simulink model "sm_car"  (R2025b)
settings: Solver=ode23t  StartTime=0.0  StopTime=100  MaxStep=0.4  RelTol=1e-3  AbsTol=1e-3  EnableMultiTasking=on
PreLoadFcn:
  | % Due to usability issue in Repeating Sequence block
  | warning('off','Simulink:Masking:Invalid');
  | 
  | % Eliminate unnecessary warnings in inactive variants
  | % Warnings generated only if you click through inactive variant
  | warning('off','MATLAB:nonExistentField');
  | warning('off','Simulink:Parameters:BlkParamUndefined');
PostLoadFcn:
  | set_param([bdroot '/Vehicle'],'popup_trailer','Off')
  | warning('off','sm:sli:setup:compile:LocalSolverNotSupported')
  | %sm_car_config_maneuver(bdroot,'WOT Braking');
  | sm_car_config_vehicle(bdroot,'false');
  | sm_car_config_logging(bdroot);
InitFcn:
  | sm_car_config_camera;
  | Vehicle = sm_car_vehcfg_checkConfig(Vehicle);
  | sm_car_check_tire_model(bdroot);
StartFcn:
  | tic;
StopFcn:
  | Elapsed_Sim_Time = toc;
  | % disp(['Elapsed Sim Time = ' num2str(Elapsed_Sim_Time)]);
undefined symbols (not defined in the file): Axle1D, AxleIn, Camera, Control, Driver, Init, Maneuver, Pedal, Scene, ShaftL1, ShaftL2, ShaftR1, ShaftR2, Visual, X, xy_data_car_side, Y, Z
libraries: sm_lib x255, fl_lib x191, nesl_utility x149, simulink x23, sdl_lib x14, simulink_extras x8, SimscapeFluids_lib x7, Scene_Utilities x6, Tire_1x2x x4, ee_lib x3, Linkage x2, fuzblock x1
(part 6 of 19)

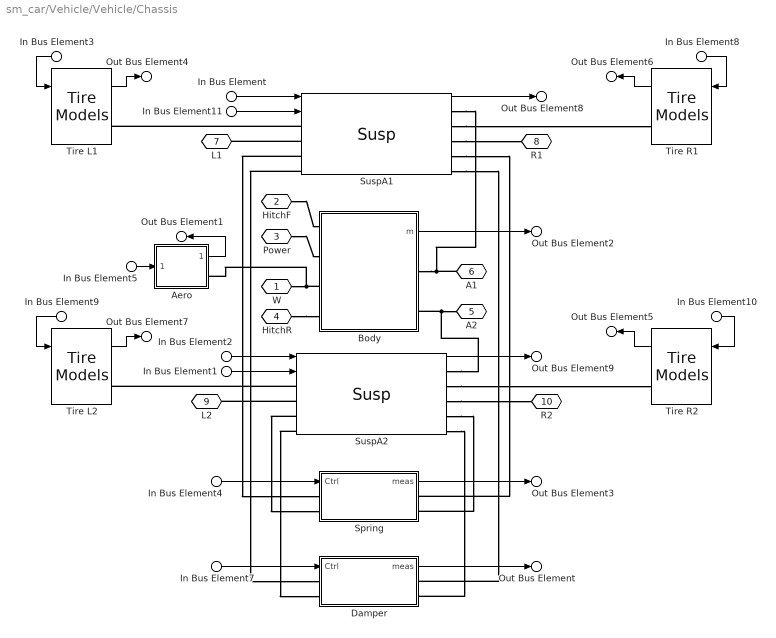
== system sm_car/Vehicle/Vehicle/Chassis ==
  In Bus Element11 : Inport  PortName=DrvBus
  In Bus Element1 : Inport  PortName=DrvBus
  In Bus Element3 : Inport  Port=2  PortName=RdBus  Element=L1
  In Bus Element8 : Inport  Port=2  PortName=RdBus  Element=R1
  In Bus Element10 : Inport  Port=2  PortName=RdBus  Element=R2
  In Bus Element9 : Inport  Port=2  PortName=RdBus  Element=L2
  In Bus Element5 : Inport  Port=2  PortName=RdBus  Element=fWindCar
  In Bus Element7 : Inport  Port=3  PortName=CtrlBus  Element=Damper
  In Bus Element : Inport  Port=3  PortName=CtrlBus  Element=SuspA1
  In Bus Element4 : Inport  Port=3  PortName=CtrlBus  Element=Spring
  In Bus Element2 : Inport  Port=3  PortName=CtrlBus  Element=SuspA2
  Aero : Subsystem  mask(Aerodynamic Load (Drag, Lift)){CL=Chassis.Aero.CL.Value, CD=Chassis.Aero.CD.Value, rho=Chassis.Aero.rho_air.Value, A=Chassis.Aero.ARef.Value, sCentreOfPressure=Chassis.Aero.sPressureCentre.Value, clr_hp=Visual.hp.clr, opc_hp=Visual.hp.opc, rad_hp=Visual.hp.rad}
      mask prompts: CL "Lift Coeff (-)"; CD "Drag Coeff (-)"; rho "Air Density (kg/m^3)"; A "Reference Area (m^2)"; sCentreOfPressure "Centre of Pressure [xyz] (m)"; clr_hp "Color [RGB]"; opc_hp "Opacity (0-1)"; rad_hp "Radius (m)"
      mask help: Models lift and drag on vehicle.
      mask TypeOptions clr_hp:
      | Vis
      | Center of Pressure/GraphicDiffuseColor
      mask TypeOptions opc_hp:
      | Vis
      | Center of Pressure/GraphicOpacity
      mask TypeOptions rad_hp:
      | Vis
      | Center of Pressure/SphereRadius
      mask DialogControl conv_vis Prompt: Visualization
  Body : Subsystem  mask(Body){hp_mount_a1=Chassis.Body.sAxle1.Value, hp_mount_a2=Chassis.Body.sAxle2.Value, hp_mount_power=Chassis.Body.sPower.Value, hp_chassis_cg=Chassis.Body.sCG.Value, hp_mount_hitchf=Chassis.Body.sHitchF.Value, hp_mount_hitchr=Chassis.Body.sHitchR.Value, chassis_mass=Chassis.Body.m.Value, chassis_inertia=Chassis.Body.J.Value, clr_chassis_hp_cg=Visual.hp.clr, opc_chassis_hp_cg=Visual.hp.opc, size_chassis_hp_cg=Visual.hp.rad, BodyGeometry=Chassis.Body.BodyGeometry, BodyLoad=Chassis.Body.BodyLoad}
      mask prompts: hp_mount_power "HP Power [xyz] (m)"; hp_chassis_cg "Chassis CG [xyz] (m)"; hp_mount_hitchf "Hitch Front [xyz] (m)"; hp_mount_hitchr "Hitch Rear [xyz] (m)"; chassis_mass "Mass (kg)"; chassis_inertia "Inertia [Ixx Iyy Izz]"; BodyGeometry "BodyGeometry (structure)"; BodyLoad "BodyLoad (structure)"
      mask help: Vehicle body mass, inertia, and geometry.
      mask TypeOptions hp_mount_a1:
      | Transform
      | Mount A1/TranslationCartesianOffset
      mask TypeOptions hp_mount_a2:
      | Transform
      | Mount A2/TranslationCartesianOffset
      mask TypeOptions hp_mount_power:
      | Transform
      | Power Mount/TranslationCartesianOffset
      mask TypeOptions hp_chassis_cg:
      | Transform
      | Body CG/TranslationCartesianOffset
      mask TypeOptions hp_mount_hitchf:
      | Transform
      | Front Hitch/TranslationCartesianOffset
      mask TypeOptions hp_mount_hitchr:
      | Transform
      | Rear Hitch/TranslationCartesianOffset
      mask TypeOptions chassis_mass:
      | Body Mass
      | and Inertia/Mass
      mask TypeOptions chassis_inertia:
      | Body Mass
      | and Inertia/MomentsOfInertia
      mask TypeOptions clr_chassis_hp_cg:
      | Body Mass
      | and Inertia/GraphicDiffuseColor | Vis HP Mount A1/GraphicDiffuseColor | Vis HP Hitch/GraphicDiffuseColor
      mask TypeOptions opc_chassis_hp_cg:
      | Body Mass
      | and Inertia/GraphicOpacity | Vis HP Mount A1/GraphicOpacity | Vis HP Hitch/GraphicOpacity
      mask TypeOptions size_chassis_hp_cg:
      | Body Mass
      | and Inertia/SphereRadius | Vis HP Mount A1/SphereRadius | Vis HP Hitch/SphereRadius
      mask DialogControl cont_chassis Prompt: Chassis
      mask DialogControl text_chassis_mount_hp_blank Prompt: [xyz] (m)
      mask DialogControl text_chassis_a1 Prompt: Axle 1
      mask DialogControl text_chassis_a2 Prompt: Axle 2
      mask DialogControl text_chassis_hp_mount Prompt: HP Mount
      mask DialogControl cont_chassis_vis Prompt: Visualization
      mask DialogControl text_chassis_vis_clr Prompt: Color [RGB]
      mask DialogControl text_chassis_vis_opc Prompt: Opacity (0-1)
      mask DialogControl text_chassis_vis_size Prompt: Size [xyz] (m)
      mask DialogControl text_chassis_vis_hp Prompt: Hardpoints
      mask DialogControl cont_body_geometry Prompt: Body
      mask Display:
      | % Get image from BodyGeometry.class
      | % (active choice for Body Geometry subsystem)
      | temp_veh_bg_class = lower(get_param([gcb '/Body Geometry'],'LabelModeActiveChoice'));
      | 
      | imagestr = (['sm_car_body_' temp_veh_bg_class '.png']);
      | if(~exist(imagestr))
      |     imagestr = ['sm_car_body_default.png'];
      | end
      | 
      | image(imagestr);
  Damper : Subsystem  Tag=PublishSubsystem  Variant=on  VariantControlMode=label  VariantControl=Variant1  LabelModeActiveChoice=Independent  mask(Variants for Dampers){Damper=Chassis.Damper, VariantLabel=Chassis.Damper.class.Value}
      mask prompts: Damper "Damper Parameters"; VariantLabel "Variant Label"
      mask help: Select option and provide parameters for left and right dampers on two axles. Option is chosen by string provided in Variant Label. The parameters for the selected option is contained in Dampers data structure.
      mask init:
      | curblk = gcb;
      | 
      | % Set variant for this block 
      | set_param(curblk,'LabelModeActiveChoice',VariantLabel);
      settings: AttributesFormatString=%<ActiveVariant>
      mask Display:
      | if(strcmp(get_param(gcb,'LabelModeActiveChoice'),'None'))
      |     disp(' ');
      | else
      |     image('sm_car_vehicle_chassis_damper_IMAGE.png');
      | end
  Spring : Subsystem  Tag=PublishSubsystem  Variant=on  VariantControlMode=label  VariantControl=Variant1  LabelModeActiveChoice=Independent  mask(Variants for Springs){Spring=Chassis.Spring, VariantLabel=Chassis.Spring.class.Value}
      mask prompts: Spring "Spring Parameters"; VariantLabel "Variant Label"
      mask help: Select option and provide parameters for left and right springs on two axles. Option is chosen by string provided in Variant Label. The parameters for the selected option is contained in Springs data structure.
      mask init:
      | curblk = gcb;
      | 
      | % Set variant for this block 
      | set_param(curblk,'LabelModeActiveChoice',VariantLabel);
      settings: AttributesFormatString=%<ActiveVariant>
      mask Display:
      | if(strcmp(get_param(gcb,'LabelModeActiveChoice'),'None'))
      |     disp(' ');
      | else
      |     image('sm_car_vehicle_chassis_spring_IMAGE.png');
      | end
  SuspA1 : Linkage/Susp  VariantControl=Variant1  LabelModeActiveChoice=Linkage  Susp=Chassis.SuspA1  Init=Init.Axle1  VariantLabel=Chassis.SuspA1.class.Value
      settings: AttributesFormatString=%<LabelModeActiveChoice>
  SuspA2 : Linkage/Susp  VariantControl=Variant1  LabelModeActiveChoice=Linkage  Susp=Chassis.SuspA2  Init=Init.Axle2  VariantLabel=Chassis.SuspA2.class.Value
      settings: AttributesFormatString=%<LabelModeActiveChoice>
  Tire L1 : Tire_1x2x/Tire Models  Tag=PublishSubsystem  VariantControl=Variant1  LabelModeActiveChoice=MFEval  popup_leftRight=Left  tir_index=veh_index  Tire=Chassis.Tire  VariantLabel=Chassis.Tire.class.Value
      settings: AttributesFormatString=%<ActiveVariant>
  Tire L2 : Tire_1x2x/Tire Models  Tag=PublishSubsystem  VariantControl=Variant1  LabelModeActiveChoice=MFEval  popup_leftRight=Left  tir_index=veh_index+10  Tire=Chassis.Tire  VariantLabel=Chassis.Tire.class.Value
      settings: AttributesFormatString=%<ActiveVariant>
  Tire R1 : Tire_1x2x/Tire Models  Tag=PublishSubsystem  VariantControl=Variant1  LabelModeActiveChoice=MFEval  popup_leftRight=Right  tir_index=veh_index+4  Tire=Chassis.Tire  VariantLabel=Chassis.Tire.class.Value
      settings: AttributesFormatString=%<ActiveVariant>
  Tire R2 : Tire_1x2x/Tire Models  Tag=PublishSubsystem  VariantControl=Variant1  LabelModeActiveChoice=MFEval  popup_leftRight=Right  tir_index=veh_index+14  Tire=Chassis.Tire  VariantLabel=Chassis.Tire.class.Value
      settings: AttributesFormatString=%<ActiveVariant>
  W : PMIOPort  Side=Right
  HitchF : PMIOPort  Port=2  Side=Right
  Power : PMIOPort  Port=3  Side=Right
  HitchR : PMIOPort  Port=4  Side=Left
  A2 : PMIOPort  Port=5  Side=Right
  A1 : PMIOPort  Port=6  Side=Left
  L1 : PMIOPort  Port=7  Side=Left
  R1 : PMIOPort  Port=8  Side=Right
  L2 : PMIOPort  Port=9  Side=Left
  R2 : PMIOPort  Port=10  Side=Right
  Out Bus Element4 : Outport  VectorParamsAs1DForOutWhenUnconnected=off  PortName=VehBus  Element=WhlL1
  Out Bus Element6 : Outport  VectorParamsAs1DForOutWhenUnconnected=off  PortName=VehBus  Element=WhlR1
  Out Bus Element5 : Outport  VectorParamsAs1DForOutWhenUnconnected=off  PortName=VehBus  Element=WhlR2
  Out Bus Element7 : Outport  VectorParamsAs1DForOutWhenUnconnected=off  PortName=VehBus  Element=WhlL2
  Out Bus Element1 : Outport  VectorParamsAs1DForOutWhenUnconnected=off  PortName=VehBus  Element=Aero
  Out Bus Element : Outport  VectorParamsAs1DForOutWhenUnconnected=off  PortName=VehBus  Element=Damper
  Out Bus Element3 : Outport  VectorParamsAs1DForOutWhenUnconnected=off  PortName=VehBus  Element=Spring
  Out Bus Element8 : Outport  VectorParamsAs1DForOutWhenUnconnected=off  PortName=VehBus  Element=SuspA1
  Out Bus Element9 : Outport  VectorParamsAs1DForOutWhenUnconnected=off  PortName=VehBus  Element=SuspA2
  Out Bus Element2 : Outport  VectorParamsAs1DForOutWhenUnconnected=off  PortName=VehBus  Element=Body
  wires:
  Body/1(m) -> Out Bus Element2/1
  In Bus Element5/1 -> Aero/1(fWind)
  Aero/1(meas) -> Out Bus Element1/1
  In Bus Element4/1 -> Spring/1("Ctrl ")
  In Bus Element7/1 -> Damper/1("Ctrl ")
  In Bus Element2/1 -> SuspA2/1
  SuspA2/1 -> Out Bus Element9/1
  In Bus Element1/1 -> SuspA2/2
  In Bus Element/1 -> SuspA1/1
  SuspA1/1 -> Out Bus Element8/1
  In Bus Element11/1 -> SuspA1/2
  Tire R2/1 -> Out Bus Element5/1
  In Bus Element9/1 -> Tire L2/1
  Tire L1/1 -> Out Bus Element4/1
  In Bus Element8/1 -> Tire R1/1
  Tire L2/1 -> Out Bus Element7/1
  In Bus Element10/1 -> Tire R2/1
  Tire R1/1 -> Out Bus Element6/1
  In Bus Element3/1 -> Tire L1/1
  Damper/1(" meas") -> Out Bus Element/1
  Spring/1(" meas") -> Out Bus Element3/1
  connections:
  HitchR/RConn1 -- Body/LConn4
  Power/RConn1 -- Body/LConn2
  SuspA2/RConn5 -- Damper/RConn2
  SuspA2/LConn4 -- Damper/LConn2
  SuspA2/RConn4 -- Spring/RConn2
  SuspA2/LConn3 -- Spring/LConn2
  SuspA2/RConn3 -- R2/RConn1
  SuspA2/LConn2 -- L2/RConn1
  SuspA2/RConn2 -- Tire R2/RConn1
  SuspA2/LConn1 -- Tire L2/RConn1
  SuspA1/RConn5 -- Damper/RConn1
  SuspA1/LConn4 -- Damper/LConn1
  SuspA1/RConn4 -- Spring/RConn1
  SuspA1/LConn3 -- Spring/LConn1
  Body/RConn1 -- SuspA1/RConn1 -- A1/RConn1
  SuspA1/LConn1 -- Tire L1/RConn1
  SuspA1/RConn2 -- Tire R1/RConn1
  SuspA1/RConn3 -- R1/RConn1
  SuspA1/LConn2 -- L1/RConn1
  A2/RConn1 -- SuspA2/RConn1 -- Body/RConn2
  W/RConn1 -- Aero/RConn1 -- Body/LConn3
  HitchF/RConn1 -- Body/LConn1

== system sm_car/Vehicle/Vehicle/Powertrain ==
  CtrlD : Inport
  CtrlP : Inport  Port=2
  VehB : Inport  Port=3
  Driveline : Subsystem  Tag=PublishSubsystem  Variant=on  VariantControlMode=label  VariantControl=Shaft  LabelModeActiveChoice=L2_R2  mask(Variants for Driveline){Driveline=Powertrain.Driveline, VariantLabel=Powertrain.Driveline.class.Value}
      mask prompts: Driveline "Driveline Parameters"; VariantLabel "Variant Label"
      mask help: Select option and provide parameters for driveline. Option is chosen by string provided in Variant Label. The parameters for the selected option are contained in Driveline data structure.
      mask init:
      | curblk = gcb;
      | 
      | % Set variant for this block 
      | set_param(curblk,'LabelModeActiveChoice',VariantLabel);
      settings: AttributesFormatString=%<ActiveVariant>
      mask Help: web('sm_car_doc_driveline.html');
  Power : Subsystem  Variant=on  VariantControlMode=label  VariantControl=Variant1  LabelModeActiveChoice=Electric_L2_R2  mask(Variants for Power){Power=Powertrain.Power, VariantLabel=Powertrain.Power.class.Value}
      mask prompts: Power "Power Parameters"; VariantLabel "Variant Label"
      mask help: Select option and provide parameters for power system (energy storage and actuator). Option is chosen by string provided in Variant Label. The parameters for the selected option are contained in Power data structure.
      mask init:
      | curblk = gcb;
      | 
      | % Set variant for this block 
      | set_param(curblk,'LabelModeActiveChoice',VariantLabel);
      settings: AttributesFormatString=%<ActiveVariant>
  FA : PMIOPort  Side=Left
  Ref : PMIOPort  Port=2  Side=Right
  RA : PMIOPort  Port=3  Side=Right
  R1 : PMIOPort  Port=4  Side=Right
  L1 : PMIOPort  Port=5  Side=Left
  L2 : PMIOPort  Port=6  Side=Left
  R2 : PMIOPort  Port=7  Side=Right
  OutD : Outport  VectorParamsAs1DForOutWhenUnconnected=off
  OutP : Outport  Port=2  VectorParamsAs1DForOutWhenUnconnected=off
  wires:
  Driveline/1(OutD) -> OutD/1
  CtrlD/1 -> Driveline/1(CtrlBus)
  Power/1(OutP) -> OutP/1
  CtrlP/1 -> Power/1(CtrlBus)
  VehB/1 -> Power/2(VehBus)
  connections:
  Driveline/LConn1 -- FA/RConn1
  Ref/RConn1 -- Power/RConn1
  Driveline/RConn1 -- RA/RConn1
  Driveline/LConn4 -- Power/LConn1
  Driveline/LConn2 -- L1/RConn1
  Driveline/RConn2 -- R1/RConn1
  Driveline/RConn3 -- R2/RConn1
  Driveline/LConn3 -- L2/RConn1

== system sm_car/Vehicle/Vehicle Constraint/No Constraint ==
  F : PMIOPort  Side=Right
  B : PMIOPort  Port=2  Side=Left

== system sm_car/Visualization/Unreal/Animation Off ==
  xyz : Inport
  rpy : Inport  Port=2
  ws : Inport  Port=3
  aCamber : Inport  Port=4
  aSteerWheel : Inport  Port=5
  Terminator{,1..4} (5 alike) : Terminator
  wires:
  rpy/1 -> Terminator1/1
  aSteerWheel/1 -> Terminator4/1
  aCamber/1 -> Terminator3/1
  xyz/1 -> Terminator/1
  ws/1 -> Terminator2/1

== system sm_car/World/Mechanism Configuration/Constant Gravity ==
  MechanismConfiguration : sm_lib/Utilities/Mechanism Configuration  UniformGravity=Constant  GravityVector=GravityVector  GravityVectorUnits=m/s^2  LinearizationDelta=0.001  JointModeTransitionNonlinearIterations=2
  C : PMIOPort  Side=Right
  connections:
  MechanismConfiguration/RConn1 -- C/RConn1

== system sm_car/World/Scene/CRG Hockenheim ==
  Finish Line : Subsystem  mask{post_h=geometry.finish_line.post.height, post_r=geometry.finish_line.post.radius, line_w=geometry.finish_line.post.separation, post_clr=geometry.finish_line.post.clr, post_opc=geometry.finish_line.post.opc, offset_xyz=geometry.finish_line.offset.xyz, offset_yaw=geometry.finish_line.offset.yaw, offset_pitch=geometry.finish_line.offset.pitch, offset_roll=geometry.finish_line.offset.roll}
      mask prompts: post_h "Post Height (m)"; post_r "Post Radius (m)"; line_w "Post Separation (m)"; post_clr "Post Color [R G B] (0-1)"; post_opc "Post Opacity (0-1)"; offset_xyz "Line Offset [x y z] (m)"; offset_yaw "Line Orientation yaw (rad)"; offset_pitch "Line Orientation pitch (rad)"; offset_roll "Line Orientation roll (rad)"
  Ground : Ground
  STL Geometry Centerline : Subsystem  mask{stl_file=geometry.centerline.filename, stl_units=geometry.centerline.fileunits, stl_clr=geometry.centerline.clr, stl_opc=geometry.centerline.opc, stl_x=geometry.centerline.x, stl_y=geometry.centerline.y, stl_z=geometry.centerline.z, stl_yaw=geometry.centerline.yaw, stl_pitch=geometry.centerline.pitch, stl_roll=geometry.centerline.roll}
      mask prompts: stl_file "CAD File"; stl_units "Units"; stl_clr "Color [R G B]"; stl_opc "Opacity (0-1)"; stl_x "Offset x (m)"; stl_y "Offset y (m)"; stl_z "Offset z (m)"; stl_yaw "Offset yaw (rad)"; stl_pitch "Offset pitch (rad)"; stl_roll "Offset roll (rad)"
      mask init:
      | set_param([gcb '/Geometry'],'ExtGeomFileName',stl_file);
      | set_param([gcb '/Geometry'],'ExtGeomFileUnits',stl_units);
  STL Geometry Road : Subsystem  mask{stl_file=geometry.filename, stl_units=geometry.fileunits, stl_clr=geometry.clr, stl_opc=geometry.opc, stl_x=geometry.x, stl_y=geometry.y, stl_z=geometry.z, stl_yaw=geometry.yaw, stl_pitch=geometry.pitch, stl_roll=geometry.roll}
      mask prompts: stl_file "CAD File"; stl_units "Units"; stl_clr "Color [R G B]"; stl_opc "Opacity (0-1)"; stl_x "Offset x (m)"; stl_y "Offset y (m)"; stl_z "Offset z (m)"; stl_yaw "Offset yaw (rad)"; stl_pitch "Offset pitch (rad)"; stl_roll "Offset roll (rad)"
      mask init:
      | set_param([gcb '/Geometry'],'ExtGeomFileName',stl_file);
      | set_param([gcb '/Geometry'],'ExtGeomFileUnits',stl_units);
  W : PMIOPort  Side=Left
  Obs : Outport  VectorParamsAs1DForOutWhenUnconnected=off
  wires:
  Ground/1 -> Obs/1
  connections:
  STL Geometry Centerline/RConn1 -- Finish Line/LConn1 -- W/RConn1 -- STL Geometry Road/RConn1

== system sm_car/World/Scene/CRG Hockenheim F ==
  Finish Line : Subsystem  mask{post_h=geometry.finish_line.post.height, post_r=geometry.finish_line.post.radius, line_w=geometry.finish_line.post.separation, post_clr=geometry.finish_line.post.clr, post_opc=geometry.finish_line.post.opc, offset_xyz=geometry.finish_line.offset.xyz, offset_yaw=geometry.finish_line.offset.yaw, offset_pitch=geometry.finish_line.offset.pitch, offset_roll=geometry.finish_line.offset.roll}
      mask prompts: post_h "Post Height (m)"; post_r "Post Radius (m)"; line_w "Post Separation (m)"; post_clr "Post Color [R G B] (0-1)"; post_opc "Post Opacity (0-1)"; offset_xyz "Line Offset [x y z] (m)"; offset_yaw "Line Orientation yaw (rad)"; offset_pitch "Line Orientation pitch (rad)"; offset_roll "Line Orientation roll (rad)"
  Ground : Ground
  STL Geometry Centerline : Subsystem  mask{stl_file=geometry.centerline.filename, stl_units=geometry.centerline.fileunits, stl_clr=geometry.centerline.clr, stl_opc=geometry.centerline.opc, stl_x=geometry.centerline.x, stl_y=geometry.centerline.y, stl_z=geometry.centerline.z, stl_yaw=geometry.centerline.yaw, stl_pitch=geometry.centerline.pitch, stl_roll=geometry.centerline.roll}
      mask prompts: stl_file "CAD File"; stl_units "Units"; stl_clr "Color [R G B]"; stl_opc "Opacity (0-1)"; stl_x "Offset x (m)"; stl_y "Offset y (m)"; stl_z "Offset z (m)"; stl_yaw "Offset yaw (rad)"; stl_pitch "Offset pitch (rad)"; stl_roll "Offset roll (rad)"
      mask init:
      | set_param([gcb '/Geometry'],'ExtGeomFileName',stl_file);
      | set_param([gcb '/Geometry'],'ExtGeomFileUnits',stl_units);
  STL Geometry Road : Subsystem  mask{stl_file=geometry.filename, stl_units=geometry.fileunits, stl_clr=geometry.clr, stl_opc=geometry.opc, stl_x=geometry.x, stl_y=geometry.y, stl_z=geometry.z, stl_yaw=geometry.yaw, stl_pitch=geometry.pitch, stl_roll=geometry.roll}
      mask prompts: stl_file "CAD File"; stl_units "Units"; stl_clr "Color [R G B]"; stl_opc "Opacity (0-1)"; stl_x "Offset x (m)"; stl_y "Offset y (m)"; stl_z "Offset z (m)"; stl_yaw "Offset yaw (rad)"; stl_pitch "Offset pitch (rad)"; stl_roll "Offset roll (rad)"
      mask init:
      | set_param([gcb '/Geometry'],'ExtGeomFileName',stl_file);
      | set_param([gcb '/Geometry'],'ExtGeomFileUnits',stl_units);
  W : PMIOPort  Side=Left
  Obs : Outport  VectorParamsAs1DForOutWhenUnconnected=off
  wires:
  Ground/1 -> Obs/1
  connections:
  STL Geometry Centerline/RConn1 -- Finish Line/LConn1 -- W/RConn1 -- STL Geometry Road/RConn1

== system sm_car/World/Scene/Double Lane Change ==
  Cones Double Lane Change : Scene_Utilities/Cones Double Lane Change  lane_width=cones.lane_width  lane_separation=cones.lane_lateral_offset  start_lane_a=cones.lane_a_offset  A1_to_A5=cones.lane_a_length  A_to_B_x=cones.gap_a_to_b  B1_to_B5=cones.lane_b_length  B_to_C_x=cones.gap_b_to_c  C1_to_C5=cones.lane_c_length  height=cones.height  baseThickness=cones.base_thickness  baseWidth=cones.base_width  coneBaseDiameter=cones.bottom_diameter  coneTopDiameter=cones.top_diameter  reflectiveStripHeight=cones.strip_height  coneColor=cones.clr  reflectiveStripColor=cones.strip_clr
  Dashes : Scene_Utilities/Dashes  dash_pitch=dashes.pitch  num_dashes=dashes.num  dash_l=dashes.l  dash_h=dashes.h  dash_w=dashes.w  thickness_base=dashes.base_h  dash_clr=dashes.clr  dash_opc=dashes.opc
  Ground : Ground
  Road : Scene_Utilities/Patch Rectangle  gp_l=road.l  gp_w=road.w  gp_h=road.h  gp_clr=road.clr  gp_opc=road.opc
  Transform Cones : sm_lib/Frames and Transforms/Rigid Transform  RotationMethod=None  FollAlignAxisA=+X  BaseAlignAxisA=+Y  FollAlignAxisB=+Y  BaseAlignAxisB=+Z  RotationStandardAxis=+Z  RotationAngle=0.0  RotationAngleUnits=deg  RotationArbitraryAxis=[0 0 1]  RotationSequenceAxes=FollowerAxes  RotationSequence=XYX  RotationSequenceAngles=[0 0 0]  RotationSequenceAnglesUnits=deg  RotationMatrix=[1 0 0; 0 1 0; 0 0 1]  Quaternion=[1 0 0 0]  TranslationMethod=StandardAxis  TranslationCartesianOffset=[0 0 0]  TranslationCartesianOffsetUnits=m  TranslationStandardAxis=-X  TranslationStandardOffset=road.l/2  TranslationStandardOffsetUnits=m  TranslationROffset=0  TranslationROffsetUnits=m  TranslationThetaOffset=0  TranslationThetaOffsetUnits=deg  TranslationZOffset=0  TranslationZOffsetUnits=m
  Transform Road : sm_lib/Frames and Transforms/Rigid Transform  RotationMethod=RotationSequence  FollAlignAxisA=+X  BaseAlignAxisA=+Y  FollAlignAxisB=+Y  BaseAlignAxisB=+Z  RotationStandardAxis=+Z  RotationAngle=0.0  RotationAngleUnits=deg  RotationArbitraryAxis=[0 0 1]  RotationSequenceAxes=BaseAxes  RotationSequence=ZYX  RotationSequenceAngles=[road.yaw road.pitch road.roll]  RotationSequenceAnglesUnits=rad  RotationMatrix=[1 0 0; 0 1 0; 0 0 1]  Quaternion=[1 0 0 0]  TranslationMethod=Cartesian  TranslationCartesianOffset=[road.x road.y road.z]  TranslationCartesianOffsetUnits=m  TranslationStandardAxis=+Z  TranslationStandardOffset=0  TranslationStandardOffsetUnits=m  TranslationROffset=0  TranslationROffsetUnits=m  TranslationThetaOffset=0  TranslationThetaOffsetUnits=deg  TranslationZOffset=0  TranslationZOffsetUnits=m
  W : PMIOPort  Side=Left
  Obs : Outport  VectorParamsAs1DForOutWhenUnconnected=off
  wires:
  Ground/1 -> Obs/1
  connections:
  W/RConn1 -- Transform Road/LConn1
  Dashes/LConn1 -- Road/RConn1 -- Transform Cones/LConn1 -- Transform Road/RConn1
  Cones Double Lane Change/LConn1 -- Transform Cones/RConn1

== system sm_car/World/Scene/Double Lane Change ISO3888 ==
  Cones Double Lane Change : Scene_Utilities/Cones Double Lane Change  lane_width=cones.lane_width  lane_separation=cones.lane_lateral_offset  start_lane_a=cones.lane_a_offset  A1_to_A5=cones.lane_a_length  A_to_B_x=cones.gap_a_to_b  B1_to_B5=cones.lane_b_length  B_to_C_x=cones.gap_b_to_c  C1_to_C5=cones.lane_c_length  height=cones.height  baseThickness=cones.base_thickness  baseWidth=cones.base_width  coneBaseDiameter=cones.bottom_diameter  coneTopDiameter=cones.top_diameter  reflectiveStripHeight=cones.strip_height  coneColor=cones.clr  reflectiveStripColor=cones.strip_clr
  Dashes : Scene_Utilities/Dashes  dash_pitch=dashes.pitch  num_dashes=dashes.num  dash_l=dashes.l  dash_h=dashes.h  dash_w=dashes.w  thickness_base=dashes.base_h  dash_clr=dashes.clr  dash_opc=dashes.opc
  Ground : Ground
  Road : Scene_Utilities/Patch Rectangle  gp_l=road.l  gp_w=road.w  gp_h=road.h  gp_clr=road.clr  gp_opc=road.opc
  Transform Cones : sm_lib/Frames and Transforms/Rigid Transform  RotationMethod=None  FollAlignAxisA=+X  BaseAlignAxisA=+Y  FollAlignAxisB=+Y  BaseAlignAxisB=+Z  RotationStandardAxis=+Z  RotationAngle=0.0  RotationAngleUnits=deg  RotationArbitraryAxis=[0 0 1]  RotationSequenceAxes=FollowerAxes  RotationSequence=XYX  RotationSequenceAngles=[0 0 0]  RotationSequenceAnglesUnits=deg  RotationMatrix=[1 0 0; 0 1 0; 0 0 1]  Quaternion=[1 0 0 0]  TranslationMethod=StandardAxis  TranslationCartesianOffset=[0 0 0]  TranslationCartesianOffsetUnits=m  TranslationStandardAxis=-X  TranslationStandardOffset=road.l/2  TranslationStandardOffsetUnits=m  TranslationROffset=0  TranslationROffsetUnits=m  TranslationThetaOffset=0  TranslationThetaOffsetUnits=deg  TranslationZOffset=0  TranslationZOffsetUnits=m
  Transform Road : sm_lib/Frames and Transforms/Rigid Transform  RotationMethod=RotationSequence  FollAlignAxisA=+X  BaseAlignAxisA=+Y  FollAlignAxisB=+Y  BaseAlignAxisB=+Z  RotationStandardAxis=+Z  RotationAngle=0.0  RotationAngleUnits=deg  RotationArbitraryAxis=[0 0 1]  RotationSequenceAxes=BaseAxes  RotationSequence=ZYX  RotationSequenceAngles=[road.yaw road.pitch road.roll]  RotationSequenceAnglesUnits=rad  RotationMatrix=[1 0 0; 0 1 0; 0 0 1]  Quaternion=[1 0 0 0]  TranslationMethod=Cartesian  TranslationCartesianOffset=[road.x road.y road.z]  TranslationCartesianOffsetUnits=m  TranslationStandardAxis=+Z  TranslationStandardOffset=0  TranslationStandardOffsetUnits=m  TranslationROffset=0  TranslationROffsetUnits=m  TranslationThetaOffset=0  TranslationThetaOffsetUnits=deg  TranslationZOffset=0  TranslationZOffsetUnits=m
  W : PMIOPort  Side=Left
  Obs : Outport  VectorParamsAs1DForOutWhenUnconnected=off
  wires:
  Ground/1 -> Obs/1
  connections:
  W/RConn1 -- Transform Road/LConn1
  Dashes/LConn1 -- Road/RConn1 -- Transform Cones/LConn1 -- Transform Road/RConn1
  Cones Double Lane Change/LConn1 -- Transform Cones/RConn1

== system sm_car/World/Scene/Plane Grid ==
  Grid : Subsystem  mask{grid_x=plane.l, grid_y=plane.w, grid_z=plane.h, grid_line_width=grid.line_width, grid_num_sq_x=grid.num_sqrs_x, grid_num_sq_y=grid.num_sqrs_y, grid_clr=grid.clr, grid_opc=grid.opc}
      mask prompts: grid_x "Length (m) (Global x)"; grid_y "Width (m) (Global y)"; grid_z "Depth (m) (Global z)"; grid_line_width "Line width (m)"; grid_num_sq_x "Number of squares in x"; grid_num_sq_y "Number of squares in y"; grid_clr "Color [RGB]"; grid_opc "Opacity (0-1)"
      mask init:
      | % Derived parameters - for two perpendicular grids with num_sq-by-1 holes
      | % **Note, not num_sq_x by num_sq_y holes - better render speed with
      | % separate meshes for x and y.
      | 
      | hole_lx = (grid_x-(grid_line_width*(grid_num_sq_x+1)))/grid_num_sq_x;
      | hole_wx = (grid_y-(grid_line_width*(1+1)))/1;
      | 
      | hole_ly = (grid_y-(grid_line_width*(grid_num_sq_y+1)))/grid_num_sq_y;
      | hole_wy = (grid_x-(grid_line_width*(1+1)))/1;
  Ground : Ground
  Ground Plane : Subsystem  mask{gp_l=plane.l, gp_w=plane.w, gp_h=plane.h, gp_clr=plane.clr, gp_opc=plane.opc}
      mask prompts: gp_l "Length (m) (Global  x)"; gp_w "Width (m) (Global  y)"; gp_h "Depth (m) (Global z)"; gp_clr "Color [R G B]"; gp_opc "Opacity (0-1)"
  Transform Plane : sm_lib/Frames and Transforms/Rigid Transform  RotationMethod=None  FollAlignAxisA=+X  BaseAlignAxisA=+Y  FollAlignAxisB=+Y  BaseAlignAxisB=+Z  RotationStandardAxis=+Z  RotationAngle=0.0  RotationAngleUnits=deg  RotationArbitraryAxis=[0 0 1]  RotationSequenceAxes=FollowerAxes  RotationSequence=XYX  RotationSequenceAngles=[0 0 0]  RotationSequenceAnglesUnits=deg  RotationMatrix=[1 0 0; 0 1 0; 0 0 1]  Quaternion=[1 0 0 0]  TranslationMethod=Cartesian  TranslationCartesianOffset=[plane.x plane.y plane.z]  TranslationCartesianOffsetUnits=m  TranslationStandardAxis=+Z  TranslationStandardOffset=0  TranslationStandardOffsetUnits=m  TranslationROffset=0  TranslationROffsetUnits=m  TranslationThetaOffset=0  TranslationThetaOffsetUnits=deg  TranslationZOffset=0  TranslationZOffsetUnits=m
  W : PMIOPort  Side=Left
  Obs : Outport  VectorParamsAs1DForOutWhenUnconnected=off
  wires:
  Ground/1 -> Obs/1
  connections:
  Ground Plane/RConn1 -- Transform Plane/RConn1 -- Grid/LConn1
  Transform Plane/LConn1 -- W/RConn1

== system sm_car/World/Scene/Skidpad ==
  Circle Inner L : Subsystem  mask{circ_d=circ_in.d, circ_a1=-180, circ_a2=180, circ_w=circ_in.w, circ_h=circ_in.h, circ_clr=circ_in.clr, circ_opc=circ_in.opc}
      mask prompts: circ_d "Circle Diameter (m)"; circ_a1 "Start Angle (deg)"; circ_a2 "Finish Angle (deg)"; circ_w "Stripe Width (m)"; circ_h "Stripe Height (m)"; circ_clr "Color [RGB]"; circ_opc "Opacity (0-1)"
      mask init:
      | xy_data_circ = Extr_Data_Ring(...
      |     circ_d/2+circ_w/2,circ_d/2-circ_w/2,circ_a1, circ_a2);
  Circle Inner R : Subsystem  mask{circ_d=circ_in.d, circ_a1=-180, circ_a2=180, circ_w=circ_in.w, circ_h=circ_in.h, circ_clr=circ_in.clr, circ_opc=circ_in.opc}
      mask prompts: circ_d "Circle Diameter (m)"; circ_a1 "Start Angle (deg)"; circ_a2 "Finish Angle (deg)"; circ_w "Stripe Width (m)"; circ_h "Stripe Height (m)"; circ_clr "Color [RGB]"; circ_opc "Opacity (0-1)"
      mask init:
      | xy_data_circ = Extr_Data_Ring(...
      |     circ_d/2+circ_w/2,circ_d/2-circ_w/2,circ_a1, circ_a2);
  Circle Outer L : Subsystem  mask{circ_d=circ_out.d, circ_a1=circ_out.ang1, circ_a2=circ_out.ang2, circ_w=circ_out.w, circ_h=circ_out.h, circ_clr=circ_out.clr, circ_opc=circ_out.opc}
      mask prompts: circ_d "Circle Diameter (m)"; circ_a1 "Start Angle (deg)"; circ_a2 "Finish Angle (deg)"; circ_w "Stripe Width (m)"; circ_h "Stripe Height (m)"; circ_clr "Color [RGB]"; circ_opc "Opacity (0-1)"
      mask init:
      | xy_data_circ = Extr_Data_Ring(...
      |     circ_d/2+circ_w/2,circ_d/2-circ_w/2,circ_a1, circ_a2);
  Circle Outer R : Subsystem  mask{circ_d=circ_out.d, circ_a1=circ_out.ang1, circ_a2=circ_out.ang2, circ_w=circ_out.w, circ_h=circ_out.h, circ_clr=circ_out.clr, circ_opc=circ_out.opc}
      mask prompts: circ_d "Circle Diameter (m)"; circ_a1 "Start Angle (deg)"; circ_a2 "Finish Angle (deg)"; circ_w "Stripe Width (m)"; circ_h "Stripe Height (m)"; circ_clr "Color [RGB]"; circ_opc "Opacity (0-1)"
      mask init:
      | xy_data_circ = Extr_Data_Ring(...
      |     circ_d/2+circ_w/2,circ_d/2-circ_w/2,circ_a1, circ_a2);
  Ground : Ground
  Ground Plane : Subsystem  mask{gp_l=plane.l, gp_w=plane.w, gp_h=plane.h, gp_clr=plane.clr, gp_opc=plane.opc}
      mask prompts: gp_l "Length (m) (Global  x)"; gp_w "Width (m) (Global  y)"; gp_h "Depth (m) (Global z)"; gp_clr "Color [R G B]"; gp_opc "Opacity (0-1)"
  Transform Circle L : sm_lib/Frames and Transforms/Rigid Transform  RotationMethod=None  FollAlignAxisA=+X  BaseAlignAxisA=+Y  FollAlignAxisB=+Y  BaseAlignAxisB=+Z  RotationStandardAxis=+Z  RotationAngle=0.0  RotationAngleUnits=deg  RotationArbitraryAxis=[0 0 1]  RotationSequenceAxes=FollowerAxes  RotationSequence=XYX  RotationSequenceAngles=[0 0 0]  RotationSequenceAnglesUnits=deg  RotationMatrix=[1 0 0; 0 1 0; 0 0 1]  Quaternion=[1 0 0 0]  TranslationMethod=Cartesian  TranslationCartesianOffset=[0 circ_in.sep/2 0]  TranslationCartesianOffsetUnits=m  TranslationStandardAxis=+Z  TranslationStandardOffset=0  TranslationStandardOffsetUnits=m  TranslationROffset=0  TranslationROffsetUnits=m  TranslationThetaOffset=0  TranslationThetaOffsetUnits=deg  TranslationZOffset=0  TranslationZOffsetUnits=m
  Transform Circle R : sm_lib/Frames and Transforms/Rigid Transform  RotationMethod=None  FollAlignAxisA=+X  BaseAlignAxisA=+Y  FollAlignAxisB=+Y  BaseAlignAxisB=+Z  RotationStandardAxis=+Z  RotationAngle=0.0  RotationAngleUnits=deg  RotationArbitraryAxis=[0 0 1]  RotationSequenceAxes=FollowerAxes  RotationSequence=XYX  RotationSequenceAngles=[0 0 0]  RotationSequenceAnglesUnits=deg  RotationMatrix=[1 0 0; 0 1 0; 0 0 1]  Quaternion=[1 0 0 0]  TranslationMethod=Cartesian  TranslationCartesianOffset=[0 -circ_in.sep/2 0]  TranslationCartesianOffsetUnits=m  TranslationStandardAxis=+Z  TranslationStandardOffset=0  TranslationStandardOffsetUnits=m  TranslationROffset=0  TranslationROffsetUnits=m  TranslationThetaOffset=0  TranslationThetaOffsetUnits=deg  TranslationZOffset=0  TranslationZOffsetUnits=m
  Transform Orient OuterL : sm_lib/Frames and Transforms/Rigid Transform  RotationMethod=StandardAxis  FollAlignAxisA=+X  BaseAlignAxisA=+Y  FollAlignAxisB=+Y  BaseAlignAxisB=+Z  RotationStandardAxis=+Z  RotationAngle=90  RotationAngleUnits=deg  RotationArbitraryAxis=[0 0 1]  RotationSequenceAxes=FollowerAxes  RotationSequence=XYX  RotationSequenceAngles=[0 0 0]  RotationSequenceAnglesUnits=deg  RotationMatrix=[1 0 0; 0 1 0; 0 0 1]  Quaternion=[1 0 0 0]  TranslationMethod=None  TranslationCartesianOffset=[0 0 0]  TranslationCartesianOffsetUnits=m  TranslationStandardAxis=+Z  TranslationStandardOffset=0  TranslationStandardOffsetUnits=m  TranslationROffset=0  TranslationROffsetUnits=m  TranslationThetaOffset=0  TranslationThetaOffsetUnits=deg  TranslationZOffset=0  TranslationZOffsetUnits=m
  Transform Orient OuterR : sm_lib/Frames and Transforms/Rigid Transform  RotationMethod=StandardAxis  FollAlignAxisA=+X  BaseAlignAxisA=+Y  FollAlignAxisB=+Y  BaseAlignAxisB=+Z  RotationStandardAxis=+Z  RotationAngle=-90  RotationAngleUnits=deg  RotationArbitraryAxis=[0 0 1]  RotationSequenceAxes=FollowerAxes  RotationSequence=XYX  RotationSequenceAngles=[0 0 0]  RotationSequenceAnglesUnits=deg  RotationMatrix=[1 0 0; 0 1 0; 0 0 1]  Quaternion=[1 0 0 0]  TranslationMethod=None  TranslationCartesianOffset=[0 0 0]  TranslationCartesianOffsetUnits=m  TranslationStandardAxis=+Z  TranslationStandardOffset=0  TranslationStandardOffsetUnits=m  TranslationROffset=0  TranslationROffsetUnits=m  TranslationThetaOffset=0  TranslationThetaOffsetUnits=deg  TranslationZOffset=0  TranslationZOffsetUnits=m
  Transform Plane : sm_lib/Frames and Transforms/Rigid Transform  RotationMethod=None  FollAlignAxisA=+X  BaseAlignAxisA=+Y  FollAlignAxisB=+Y  BaseAlignAxisB=+Z  RotationStandardAxis=+Z  RotationAngle=0.0  RotationAngleUnits=deg  RotationArbitraryAxis=[0 0 1]  RotationSequenceAxes=FollowerAxes  RotationSequence=XYX  RotationSequenceAngles=[0 0 0]  RotationSequenceAnglesUnits=deg  RotationMatrix=[1 0 0; 0 1 0; 0 0 1]  Quaternion=[1 0 0 0]  TranslationMethod=Cartesian  TranslationCartesianOffset=[plane.x plane.y plane.z]  TranslationCartesianOffsetUnits=m  TranslationStandardAxis=+Z  TranslationStandardOffset=0  TranslationStandardOffsetUnits=m  TranslationROffset=0  TranslationROffsetUnits=m  TranslationThetaOffset=0  TranslationThetaOffsetUnits=deg  TranslationZOffset=0  TranslationZOffsetUnits=m
  W : PMIOPort  Side=Left
  Obs : Outport  VectorParamsAs1DForOutWhenUnconnected=off
  wires:
  Ground/1 -> Obs/1
  connections:
  Circle Outer L/RConn1 -- Transform Orient OuterL/RConn1
  Circle Outer R/RConn1 -- Transform Orient OuterR/RConn1
  Circle Inner R/RConn1 -- Transform Circle R/RConn1 -- Transform Orient OuterR/LConn1
  Transform Plane/RConn1 -- Ground Plane/RConn1
  Transform Circle L/LConn1 -- W/RConn1 -- Transform Plane/LConn1 -- Transform Circle R/LConn1
  Circle Inner L/RConn1 -- Transform Circle L/RConn1 -- Transform Orient OuterL/LConn1

== system sm_car/Controller/Default/Brake Control/Pedal ==
  rBrakePedal : Inport
  VehBus : Inport  Port=2
  Apply{,1..3} (4 alike) : Constant  Value=[0 1]
  Bus Creator : BusCreator  Inputs=1
  Bus Creator1 : BusCreator  Inputs=4
  Terminator : Terminator
  Terminator1 : Terminator
  Brakes : Outport  VectorParamsAs1DForOutWhenUnconnected=off
  wires:
  rBrakePedal/1 -> Terminator1/1
  Apply3/1 -> Bus Creator1/4  "R2"
  Apply2/1 -> Bus Creator1/3  "L2"
  Apply1/1 -> Bus Creator1/2  "R1"
  Apply/1 -> Bus Creator1/1  "L1"
  Bus Creator1/1 -> Bus Creator/1  "Valves"
  VehBus/1 -> Terminator/1
  Bus Creator/1 -> Brakes/1  "Brakes"

== system sm_car/Controller/FeedF_Ctrl/Brake Control/Pedal ==
  rBrakePedal : Inport
  VehBus : Inport  Port=2
  Apply{,1..3} (4 alike) : Constant  Value=[0 1]
  Bus Creator : BusCreator  Inputs=1
  Bus Creator1 : BusCreator  Inputs=4
  Terminator : Terminator
  Terminator1 : Terminator
  Brakes : Outport  VectorParamsAs1DForOutWhenUnconnected=off
  wires:
  Bus Creator/1 -> Brakes/1  "Brakes"
  VehBus/1 -> Terminator/1
  Bus Creator1/1 -> Bus Creator/1  "Valves"
  Apply/1 -> Bus Creator1/1  "L1"
  Apply1/1 -> Bus Creator1/2  "R1"
  Apply2/1 -> Bus Creator1/3  "L2"
  Apply3/1 -> Bus Creator1/4  "R2"
  rBrakePedal/1 -> Terminator1/1

== system sm_car/Controller/NoIMU/Brake Control/Pedal ==
  rBrakePedal : Inport
  VehBus : Inport  Port=2
  Apply{,1..3} (4 alike) : Constant  Value=[0 1]
  Bus Creator : BusCreator  Inputs=1
  Bus Creator1 : BusCreator  Inputs=4
  Terminator : Terminator
  Terminator1 : Terminator
  Brakes : Outport  VectorParamsAs1DForOutWhenUnconnected=off
  wires:
  Bus Creator/1 -> Brakes/1  "Brakes"
  VehBus/1 -> Terminator/1
  Bus Creator1/1 -> Bus Creator/1  "Valves"
  Apply/1 -> Bus Creator1/1  "L1"
  Apply1/1 -> Bus Creator1/2  "R1"
  Apply2/1 -> Bus Creator1/3  "L2"
  Apply3/1 -> Bus Creator1/4  "R2"
  rBrakePedal/1 -> Terminator1/1

== system sm_car/Controller/NoIMU/Power Control/Current-Torque ==
  note: modify to accomade all voltage ranges
      | only 220V now
  note: current - torque
  V : Inport
  Il : Inport  Port=2
  Ir : Inport  Port=3
  Add : Sum
  Km : Gain  Gain=Km
  Km1 : Gain  Gain=Km
  Terminator : Terminator
  Out1 : Outport
  wires:
  Il/1 -> Km1/1
  Km1/1 -> Add/1
  V/1 -> Terminator/1
  Ir/1 -> Km/1
  Add/1 -> Out1/1
  Km/1 -> Add/2

== system sm_car/Controller/NoIMU/Power Control/Slip Control ==
  VehBus : Inport
  Bus Selector : BusSelector  OutputSignals=Power.MotorL2.w,Power.MotorL2.i,Power.MotorR2.w,Power.MotorR2.i
  Constant : Constant
  Constant1 : Constant  Value=0
  I no load : Constant  Value=I0
  Product : Product
  Product1 : Product
  Relational Operator : RelationalOperator  OutDataTypeStr=boolean  RndMeth=Simplest  InputSameDT=off
  Relational Operator1 : RelationalOperator  Operator=<=  OutDataTypeStr=boolean  RndMeth=Simplest  InputSameDT=off
  Relational Operator2 : RelationalOperator  OutDataTypeStr=boolean  RndMeth=Simplest  InputSameDT=off
  Relational Operator3 : RelationalOperator  Operator=<=  OutDataTypeStr=boolean  RndMeth=Simplest  InputSameDT=off
  Switch : Switch  Criteria=u2 > Threshold  SaturateOnIntegerOverflow=off  InputSameDT=off
  Switch1 : Switch  Criteria=u2 > Threshold  SaturateOnIntegerOverflow=off  InputSameDT=off
  w no load : Constant  Value=w0
  Out1 : Outport
  Out2 : Outport  Port=2
  wires:
  VehBus/1 -> Bus Selector/1
  Bus Selector/1 -> Relational Operator/1  "<w>"
  Product/1 -> Switch/2
  Relational Operator/1 -> Product/1
  Relational Operator1/1 -> Product/2
  Relational Operator2/1 -> Product1/1
  Relational Operator3/1 -> Product1/2
  Product1/1 -> Switch1/2
  Constant1/1 -> Switch/3, Switch1/3
  Constant/1 -> Switch1/1, Switch/1
  Bus Selector/2 -> Relational Operator1/1  "<i>"
  Bus Selector/3 -> Relational Operator2/1  "<w>"
  Bus Selector/4 -> Relational Operator3/1  "<i>"
  I no load/1 -> Relational Operator1/2, Relational Operator3/2
  w no load/1 -> Relational Operator/2, Relational Operator2/2
  Switch/1 -> Out1/1
  Switch1/1 -> Out2/1

== system sm_car/Controller/Slip_Ctrl/Brake Control/Pedal ==
  rBrakePedal : Inport
  VehBus : Inport  Port=2
  Apply{,1..3} (4 alike) : Constant  Value=[0 1]
  Bus Creator : BusCreator  Inputs=1
  Bus Creator1 : BusCreator  Inputs=4
  Terminator : Terminator
  Terminator1 : Terminator
  Brakes : Outport  VectorParamsAs1DForOutWhenUnconnected=off
  wires:
  Bus Creator/1 -> Brakes/1  "Brakes"
  VehBus/1 -> Terminator/1
  Bus Creator1/1 -> Bus Creator/1  "Valves"
  Apply/1 -> Bus Creator1/1  "L1"
  Apply1/1 -> Bus Creator1/2  "R1"
  Apply2/1 -> Bus Creator1/3  "L2"
  Apply3/1 -> Bus Creator1/4  "R2"
  rBrakePedal/1 -> Terminator1/1

== system sm_car/Controller/TrqVec 4Motor/Brake Control/ABS ==
  rBrakePedal : Inport
  In Bus Element1 : Inport  Port=2  PortName=VehBus  Element=Chassis
  In Bus Element2 : Inport  Port=2  PortName=VehBus  Element=Chassis.Body.CG
  Bus Creator1 : BusCreator  Inputs=4
  Bus Creator2 : BusCreator  Inputs=1
  Bus Selector : BusSelector  OutputSignals=L1
  Bus Selector1 : BusSelector  OutputSignals=R1
  Bus Selector2 : BusSelector  OutputSignals=L2
  Bus Selector3 : BusSelector  OutputSignals=R2
  Calculate Slip : Subsystem
  Sensor : Subsystem
  Terminator : Terminator
  Valve Control L1 : Subsystem
  Valve Control L2 : Subsystem
  Valve Control R1 : Subsystem
  Valve Control R2 : Subsystem
  Vehicle Speed : Subsystem
  Brakes : Outport  VectorParamsAs1DForOutWhenUnconnected=off
  wires:
  rBrakePedal/1 -> Terminator/1
  Vehicle Speed/1(vSpdEst) -> Valve Control R2/2(vSpdEst), Valve Control L2/2(vSpdEst), Valve Control R1/2(vSpdEst), Valve Control L1/2(vSpdEst), Calculate Slip/2(VehSpdEst)
  Sensor/1(GroundSpd) -> Vehicle Speed/1(Sensors), Calculate Slip/1(WhlSpd)
  Bus Creator1/1 -> Bus Creator2/1  "Valves"
  Bus Selector2/1 -> Valve Control L2/1(Slip)  "<L2>"
  Valve Control R1/1(Valve) -> Bus Creator1/2  "R1"
  Valve Control R2/1(Valve) -> Bus Creator1/4  "R2"
  Valve Control L2/1(Valve) -> Bus Creator1/3  "L2"
  Bus Selector3/1 -> Valve Control R2/1(Slip)  "<R2>"
  Bus Selector/1 -> Valve Control L1/1(Slip)  "<L1>"
  Calculate Slip/1(Slip) -> Bus Selector3/1, Bus Selector2/1, Bus Selector1/1, Bus Selector/1
  Valve Control L1/1(Valve) -> Bus Creator1/1  "L1"
  Bus Selector1/1 -> Valve Control R1/1(Slip)  "<R1>"
  Bus Creator2/1 -> Brakes/1  "Brakes"
  In Bus Element1/1 -> Sensor/2(WhlSpd)
  In Bus Element2/1 -> Sensor/1(Body)

== system sm_car/Controller/TrqVec 4Motor/Brake Control/Pedal ==
  rBrakePedal : Inport
  VehBus : Inport  Port=2
  Apply{,1..3} (4 alike) : Constant  Value=[0 1]
  Bus Creator : BusCreator  Inputs=1
  Bus Creator1 : BusCreator  Inputs=4
  Terminator : Terminator
  Terminator1 : Terminator
  Brakes : Outport  VectorParamsAs1DForOutWhenUnconnected=off
  wires:
  rBrakePedal/1 -> Terminator1/1
  Apply3/1 -> Bus Creator1/4  "R2"
  Apply2/1 -> Bus Creator1/3  "L2"
  Apply1/1 -> Bus Creator1/2  "R1"
  Apply/1 -> Bus Creator1/1  "L1"
  Bus Creator1/1 -> Bus Creator/1  "Valves"
  VehBus/1 -> Terminator/1
  Bus Creator/1 -> Brakes/1  "Brakes"

== system sm_car/Controller/TrqVec 4Motor/Brake Control/Pressure ==
  rBrakePedal : Inport
  VehBus : Inport  Port=2
  Bus Creator : BusCreator  Inputs=4
  Gain : Gain  Gain=Vehicle.Brakes.Front.Caliper.pMax.Value
  Gain1 : Gain  Gain=Vehicle.Brakes.Front.Caliper.pMax.Value
  Gain2 : Gain  Gain=Vehicle.Brakes.Rear.Caliper.pMax.Value
  Gain3 : Gain  Gain=Vehicle.Brakes.Rear.Caliper.pMax.Value
  Terminator : Terminator
  Brakes : Outport  VectorParamsAs1DForOutWhenUnconnected=off
  wires:
  rBrakePedal/1 -> Gain/1, Gain1/1, Gain3/1, Gain2/1
  VehBus/1 -> Terminator/1
  Bus Creator/1 -> Brakes/1  "Brakes"
  Gain/1 -> Bus Creator/1  "pBrakeL1"
  Gain1/1 -> Bus Creator/2  "pBrakeR1"
  Gain2/1 -> Bus Creator/3  "pBrakeL2"
  Gain3/1 -> Bus Creator/4  "pBrakeR2"

== system sm_car/Controller/TrqVec 4Motor/Power_TqVec/Torque Vectoring ==
  trqA2 : Inport
  vx : Inport  Port=2
  aSteerWheel : Inport  Port=3
  wL2 : Inport  Port=4
  wR2 : Inport  Port=5
  nYaw : Inport  Port=6
  rBrake : Inport  Port=7
  Accel Torque Request : Subsystem
  Calculate Torque Split : MATLAB Function  TreatAsAtomicUnit=on
  Compare To Constant1 : simulink/Logic and Bit Operations/Compare To Constant  relop=<  const=.01  OutDataTypeStr=boolean
  Data Type Conversion : DataTypeConversion  SaturateOnIntegerOverflow=off  RndMeth=Floor
  Enable : Subsystem
  Gain1 : Gain  Gain=0.5
  Gain5 : Gain
  Gain6 : Gain
  Max Delta Torque : Constant  Value=max_torque_delta
  PID Controller : slpidlib/PID Controller  Controller=PID  Form=Parallel  TimeDomain=Continuous-time  UseExternalTs=off  SampleTime=-1  IntegratorMethod=Forward Euler  FilterMethod=Forward Euler  ControllerParametersSource=internal  P=P  I=I  UseKiTs=off  D=0  UseExternalDerivativeSource=off  N=1  UseFilter=on  TunerSelectOption=Transfer Function Based (PID Tuner App)  InitialConditionSource=internal  InitialConditionForIntegrator=0  InitialConditionForFilter=0  DifferentiatorICPrevScaledInput=0  ExternalReset=either  TrackingMode=off  Kt=1  LimitOutput=off  SatLimitsSource=internal  UpperSaturationLimit=inf  LowerSaturationLimit=-inf  LinearizeAsGain=on  AntiWindupMode=back-calculation  Kb=1  LimitIntegrator=off  UpperIntegratorSaturationLimit=inf  LowerIntegratorSaturationLimit=-inf  POutMin=[]  POutMax=[]  IOutMin=[]  IOutMax=[]  DOutMin=[]  DOutMax=[]  NOutMin=[]  NOutMax=[]  SumOutMin=[]  SumOutMax=[]  SaturationOutMin=[]  SaturationOutMax=[]  PParamMin=[]  PParamMax=[]  IParamMin=[]  IParamMax=[]  DParamMin=[]  DParamMax=[]  NParamMin=[]  NParamMax=[]  KbParamMin=[]  KbParamMax=[]  KtParamMin=[]  KtParamMax=[]  KbOutMin=[]  KbOutMax=[]  KtOutMin=[]  KtOutMax=[]  IntegratorOutMin=[]  IntegratorOutMax=[]  FilterOutMin=[]  FilterOutMax=[]  SumI1OutMin=[]  SumI1OutMax=[]  SumI2OutMin=[]  SumI2OutMax=[]  SumI3OutMin=[]  SumI3OutMax=[]  SumI4OutMin=[]  SumI4OutMax=[]  SumDOutMin=[]  SumDOutMax=[]  DifferentiatorOutMin=[]  DifferentiatorOutMax=[]  FilterDiffOutCoefMin=[]  FilterDiffOutCoefMax=[]  ReciprocalOutMin=[]  ReciprocalOutMax=[]  SumDenOutMin=[]  SumDenOutMax=[]  SumNumOutMin=[]  SumNumOutMax=[]  DivideOutMin=[]  DivideOutMax=[]  UdiffTsProdOutMin=[]  UdiffTsProdOutMax=[]  NTsProdOutMin=[]  NTsProdOutMax=[]  UintegralTsProdOutMin=[]  UintegralTsProdOutMax=[]  UngainTsProdOutMin=[]  UngainTsProdOutMax=[]  ClampingZeroOutDataTypeStr=Inherit: Inherit via back propagation  ClampingZeroOutMin=[]  ClampingZeroOutMax=[]  FilterDenConstantOutDataTypeStr=Inherit: Inherit via back propagation  FilterDenConstantOutMin=[]  FilterDenConstantOutMax=[]  PCopyOutDataTypeStr=Inherit: Inherit via back propagation  PCopyOutMin=[]  PCopyOutMax=[]  NCopyOutDataTypeStr=Inherit: Inherit via back propagation  NCopyOutMin=[]  NCopyOutMax=[]  IntegratorContinuousStateAttributes=''  IntegratorStateMustResolveToSignalObject=off  IntegratorRTWStateStorageClass=Auto  FilterContinuousStateAttributes=''  FilterStateMustResolveToSignalObject=off  FilterRTWStateStorageClass=Auto  ParallelPVariant=InternalParameters  IdealPVariant=Disabled  IVariant=InternalParameters  DVariant=InternalParameters  IntegratorVariant=Continuous  SatVariant=Disabled  AWVariant=Passthrough  PCopyVariant=Disabled  TRVariant=Disabled  FdbkBlocksVariant=Forward  IdealPFdbkVariant=Disabled  SatFdbkVariant=Disabled  DerivativeFilterVariant=ContFilter  NVariant=InternalParameters  NCopyVariant=Disabled  FilterICVariant=InternalICsFilter  IntegratorICVariant=InternalICs  ExternalResetVariant=ExternalReset  TRSumVariant=Passthrough  SumFdbkVariant=Disabled  SumVariant=Sum_PID  TsampFilterVariant=InternalTs  TsampNgainVariant=Passthrough  TsampIntegralVariant=Disabled_SignalSpec  ExternalSaturationOutDataTypeStr=Inherit: Same as second input  DerivativeSourceVariant=ErrorSignal  PreIntVariant=InternalPreInt
  Transfer Fcn : TransferFcn  Denominator=[0.5 1]
  Transfer Fcn1 : TransferFcn  Denominator=[.001 1]
  Transfer Fcn2 : TransferFcn  Denominator=[.001 1]
  Vehicle Slip Angle Error : Subsystem
  trqL2 : Outport  VectorParamsAs1DForOutWhenUnconnected=off
  trqR2 : Outport  Port=2  VectorParamsAs1DForOutWhenUnconnected=off
  wires:
  Compare To Constant1/1 -> Data Type Conversion/1
  Data Type Conversion/1 -> Transfer Fcn/1
  Max Delta Torque/1 -> Calculate Torque Split/2(max_delta_trq)
  nYaw/1 -> Vehicle Slip Angle Error/3(nYaw)
  Enable/1(Enable) -> Calculate Torque Split/1(enable), PID Controller/2  "Enable"
  Gain1/1 -> Calculate Torque Split/4(tq_l), Calculate Torque Split/5(tq_r)
  rBrake/1 -> Compare To Constant1/1
  Gain6/1 -> trqR2/1
  Vehicle Slip Angle Error/1(Error) -> PID Controller/1
  Calculate Torque Split/1(tq_l_out) -> Gain5/1
  Transfer Fcn/1 -> Calculate Torque Split/7(brk)
  Transfer Fcn2/1 -> Accel Torque Request/2(MotSpdR2)
  trqA2/1 -> Gain1/1
  Calculate Torque Split/2(tq_r_out) -> Gain6/1
  wR2/1 -> Transfer Fcn2/1
  PID Controller/1 -> Calculate Torque Split/6(tq_tv)
  Gain5/1 -> trqL2/1
  aSteerWheel/1 -> Enable/2(aSteerWheel), Vehicle Slip Angle Error/2(aSteerWheel)
  vx/1 -> Enable/1(vx), Vehicle Slip Angle Error/1(vx)
  Accel Torque Request/1(TrqMax) -> Calculate Torque Split/3(max_tq)
  Transfer Fcn1/1 -> Accel Torque Request/1(MotSpdL2)
  wL2/1 -> Transfer Fcn1/1
